simulink model "MultiSynapseTest"  (R2020b)
settings: Solver=ode45  StartTime=0.0  StopTime=2  RelTol=1e-3  EnableMultiTasking=on
libraries: NeuroModelerLibrary x5
settings Model: Creator=Bakhshiev  LastModifiedBy=Bakhshiev
settings DataIOCC: LimitDataPoints=on  SaveFormat=Array  SignalLoggingSaveFormat=ModelDataLogs  ReturnWorkspaceOutputs=off
settings OptimizationCC: ExpressionDepthLimit=2147483647  InitFltsAndDblsToZero=on  LifeSpan=inf
settings DebuggingCC: UnderspecifiedInitializationDetection=Classic  MergeDetectMultiDrivingBlocksExec=none  SolverPrmCheckMsg=warning  FcnCallInpInsideContextMsg=warning  StateNameClashWarn=warning  SFUnexpectedBacktrackingDiag=warning  SFNoUnconditionalDefaultTransitionDiag=warning  SFExecutionAtInitializationDiag=none  ArithmeticOperatorsInVariantConditions=warning
settings HardwareCC: ProdBitPerPointer=32  ProdBitPerSizeT=32  ProdBitPerPtrDiffT=32  ProdLargestAtomicFloat=None  ProdIntDivRoundTo=Undefined  ProdEndianess=Unspecified  ProdWordSize=32  ProdHWDeviceType=32-bit Generic
settings ModelReferenceCC: PropagateSignalLabelsOutOfModel=off
settings SFSimCC: CustomCodeUndefinedFunction=UseInterfaceOnly
settings CodeAppCC: StateflowObjectComments=on
settings GRTTargetCC: TargetLangStandard=C89/C90 (ANSI)  CombineOutputUpdateFcns=off  GRTInterface=on
settings ConfigComp: CovMetricSettings=dw  CovSaveCumulativeToWorkspaceVar=on  CovSaveSingleToWorkspaceVar=on

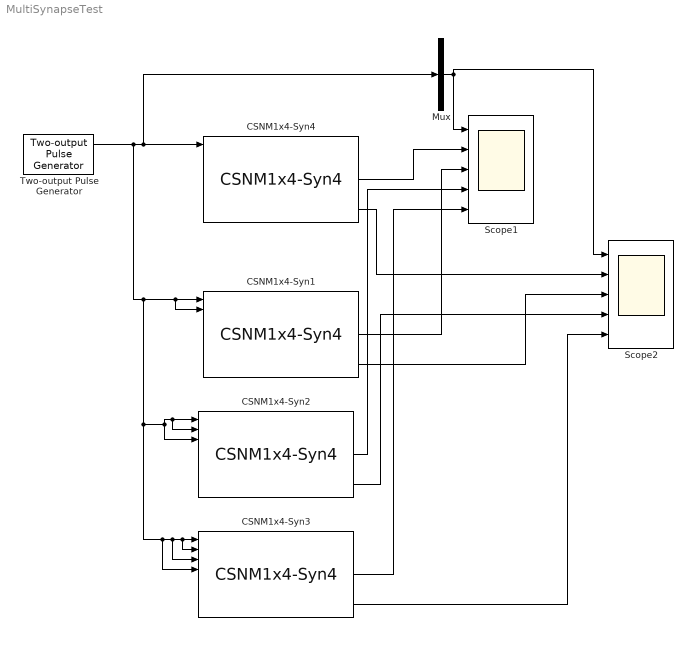
== system MultiSynapseTest ==
  CSNM1x4-Syn{1..4} (4 alike) : NeuroModelerLibrary/Sized Cells/CSNM1x4-Syn4  SystemSampleTime=-1  VariantActivationTime=update diagram  Latency=0  AutoFrameSizeCalculation=off
  Mux : Mux  Inputs=1
  Scope1 : Scope  NumInputPorts=5
  Scope2 : Scope  NumInputPorts=5
  Two-output Pulse Generator : NeuroModelerLibrary/Support/Two-output Pulse Generator  A=1  P1=200  P2=200  PW=1  ST=0.001  OOn1=0.5  OOff1=0.6  OOn2=0.8  OOff2=0.9
  wires:
  Two-output Pulse Generator/1 -> CSNM1x4-Syn4/1, Mux/1, CSNM1x4-Syn1/1, CSNM1x4-Syn1/2, CSNM1x4-Syn3/4, CSNM1x4-Syn3/3, CSNM1x4-Syn3/2, CSNM1x4-Syn3/1, CSNM1x4-Syn2/3, CSNM1x4-Syn2/1, CSNM1x4-Syn2/2
  Mux/1 -> Scope2/1, Scope1/1
  CSNM1x4-Syn4/2 -> Scope1/2
  CSNM1x4-Syn1/2 -> Scope1/3
  CSNM1x4-Syn2/2 -> Scope1/4
  CSNM1x4-Syn3/2 -> Scope1/5
  CSNM1x4-Syn4/3 -> Scope2/2
  CSNM1x4-Syn1/3 -> Scope2/3
  CSNM1x4-Syn2/3 -> Scope2/4
  CSNM1x4-Syn3/3 -> Scope2/5
